simulink model "Husky_G2G"  (R2024b)
settings: Solver=VariableStepAuto  StartTime=0.0  StopTime=inf  RelTol=1e-3
settings Model: DataDictionary=DataDictionary.sldd  Creator=charber  LastModifiedBy=tsamak
settings DebuggingCC: AlgebraicLoopMsg=none
settings ModelReferenceCC: ModelReferenceMinAlgLoopOccurrences=on

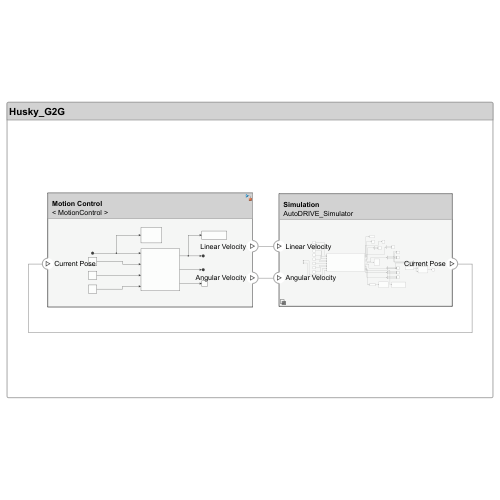
[thumbnail: Simulink's stored preview of the top-level diagram]
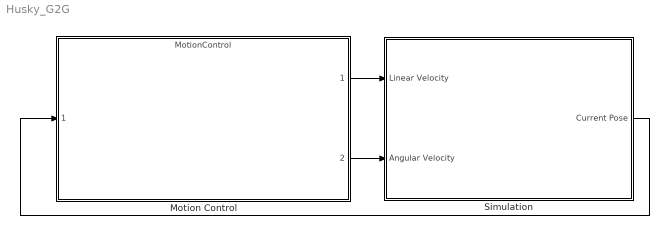
== system Husky_G2G ==
  Motion Control : ModelReference  ModelNameDialog=MotionControl  UsingDefaultArgumentValue=0,0  SimulationMode=Normal  ModelReferenceVersion=2.12
      settings: PortSchema="{\"entries\":[{\"content\":{\"headerSize\":38,\"margin\":15,\"minimumSpacing\":25,\"sides\":[{\"content\":{\"connectorIds\":[\"In1\"]},\"type\":\"ConnectorPlacement.EquallySpacedRectSide\",\"uuid\":\"c98b129e-902f-480e-b35c-0d51e818fc74\"},{\"content\":{\"connectorIds\":[\"Out1\",\"Out2\"],\"side\":\"RIGHT\"},\"type\":\"ConnectorPlacement.EquallySpacedRectSide\",\"uuid\":\"6995c358-3616-4018-88cf-5d39b6da6a01\"},{\"content\":{\"side\":\"TOP\"},\"type\":\"ConnectorPlacement.EquallySpacedRectSide\",\"uuid\":\"9fd3bced-19a7-4eda-9800-31df169afecb\"}]},\"type\":\"ConnectorPlacement.EquallySpacedConnector\",\"uuid\":\"67565f83-f33b-4056-998b-9174ff38aca6\"}],\"packageUris\":[\"http://schema.mathworks.com/mf0/Connector/R2020b\"],\"version\":\"1.0\"}"
  Simulation : Subsystem  Variant=on  VariantControlMode=label  LabelModeActiveChoice=AutoDRIVE_Simulator
      settings: PortSchema="{\"entries\":[{\"content\":{\"headerSize\":38,\"margin\":15,\"minimumSpacing\":25,\"sides\":[{\"content\":{\"connectorIds\":[\"In1\",\"In2\"]},\"type\":\"ConnectorPlacement.EquallySpacedRectSide\",\"uuid\":\"928e42ed-4929-44d9-97ae-60c1add01b45\"},{\"content\":{\"connectorIds\":[\"Out1\"],\"side\":\"RIGHT\"},\"type\":\"ConnectorPlacement.EquallySpacedRectSide\",\"uuid\":\"265edb96-fe63-44e6-ab1f-9b35c7a83ccb\"},{\"content\":{\"side\":\"TOP\"},\"type\":\"ConnectorPlacement.EquallySpacedRectSide\",\"uuid\":\"c0006a31-ac86-4900-ae15-35bc44301cb7\"},{\"content\":{\"side\":\"BOTTOM\"},\"type\":\"ConnectorPlacement.EquallySpacedRectSide\",\"uuid\":\"3ee4aa34-6775-40d9-ae3d-040d6c8ae2c4\"}]},\"type\":\"ConnectorPlacement.EquallySpacedConnector\",\"uuid\":\"c5754a81-9857-403b-bbb7-4e4b912d146f\"}],\"packageUris\":[\"http://schema.mathworks.com/mf0/Connector/R2020b\"],\"version\":\"1.0\"}"
  wires:
  Simulation/1(Current Pose) -> Motion Control/1
  Motion Control/2 -> Simulation/2(Angular Velocity)
  Motion Control/1 -> Simulation/1(Linear Velocity)

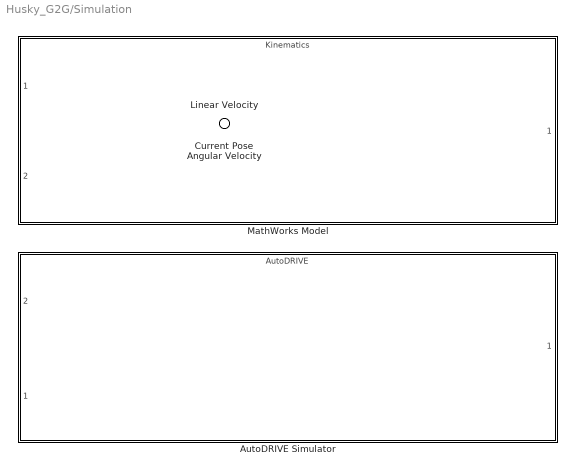
== system Husky_G2G/Simulation ==
  Linear Velocity : Inport  OutDataTypeStr=double
  Angular Velocity : Inport  Port=2  OutDataTypeStr=double
  AutoDRIVE Simulator : ModelReference  ModelNameDialog=AutoDRIVE  SimulationMode=Normal  VariantControl=AutoDRIVE_Simulator  ModelReferenceVersion=1.24
      settings: PortSchema="{\"entries\":[{\"content\":{\"headerSize\":38,\"margin\":15,\"minimumSpacing\":25,\"sides\":[{\"content\":{\"connectorIds\":[\"In2\",\"In1\"]},\"type\":\"ConnectorPlacement.EquallySpacedRectSide\",\"uuid\":\"fff1038f-badb-4c3d-a9b4-39a003bde29c\"},{\"content\":{\"connectorIds\":[\"Out1\"],\"side\":\"RIGHT\"},\"type\":\"ConnectorPlacement.EquallySpacedRectSide\",\"uuid\":\"acfb8ae9-60f1-493f-9871-3959ae422a33\"},{\"content\":{\"side\":\"TOP\"},\"type\":\"ConnectorPlacement.EquallySpacedRectSide\",\"uuid\":\"e34f200b-c261-4832-b8dd-0cbae5258d3b\"}]},\"type\":\"ConnectorPlacement.EquallySpacedConnector\",\"uuid\":\"d4137258-0861-4dce-ac93-2c30ef95f038\"}],\"packageUris\":[\"http://schema.mathworks.com/mf0/Connector/R2020b\"],\"version\":\"1.0\"}"
  MathWorks Model : ModelReference  ModelNameDialog=Kinematics.slx  SimulationMode=Normal  VariantControl=MathWorks_Model  ModelReferenceVersion=2.13
      settings: PortSchema="{\"entries\":[{\"content\":{\"headerSize\":38,\"margin\":15,\"minimumSpacing\":25,\"sides\":[{\"content\":{\"connectorIds\":[\"In1\",\"In2\"]},\"type\":\"ConnectorPlacement.EquallySpacedRectSide\",\"uuid\":\"c98b129e-902f-480e-b35c-0d51e818fc74\"},{\"content\":{\"connectorIds\":[\"Out1\"],\"side\":\"RIGHT\"},\"type\":\"ConnectorPlacement.EquallySpacedRectSide\",\"uuid\":\"6995c358-3616-4018-88cf-5d39b6da6a01\"},{\"content\":{\"side\":\"TOP\"},\"type\":\"ConnectorPlacement.EquallySpacedRectSide\",\"uuid\":\"9fd3bced-19a7-4eda-9800-31df169afecb\"}]},\"type\":\"ConnectorPlacement.EquallySpacedConnector\",\"uuid\":\"67565f83-f33b-4056-998b-9174ff38aca6\"}],\"packageUris\":[\"http://schema.mathworks.com/mf0/Connector/R2020b\"],\"version\":\"1.0\"}"
  Current Pose : Outport
